simulink model "PV_MPPT_DesktopSim"  (R2025b)
settings: Solver=ode23t  StartTime=0.0  StopTime=inf  MaxStep=1e-4  RelTol=1e-3
PreLoadFcn:
  | load('EmulatedPV_LowPowerData.mat');
  | 
  | numIrr = 10;
  | ArrayPower = ArrayCurrent.*ArrayVoltage;
InitFcn:
  | Ts = 1e-4;
  | Tc = Ts;
undefined symbols (not defined in the file): ArrayCurrent, ArrayVoltage, DiscIntNeverNeededParam, Irradiance, Tdata
libraries: fl_lib x15, nesl_utility x9, ee_lib x2, slpidlib x2, eePwmGeneratorMultilevel x1, simulink x1, eePwmGenerator x1, eePowerMeasurement x1
settings Model: Creator=mmishra  LastModifiedBy=jlesage
settings SolverCC: AlgebraicLoopSolver=TrustRegion
settings DataIOCC: ReturnWorkspaceOutputs=off
settings DebuggingCC: UnconnectedInputMsg=warning  UnconnectedOutputMsg=warning  UnconnectedLineMsg=warning  ArithmeticOperatorsInVariantConditions=warning
settings ModelReferenceCC: EnableRefExpFcnMdlSchedulingChecks=on
settings SFSimCC: SimUseLocalCustomCode=off  CustomCodeUndefinedFunction=UseInterfaceOnly
settings RTWCC: RTWUseLocalCustomCode=off  GPUComputeCapability=3.5

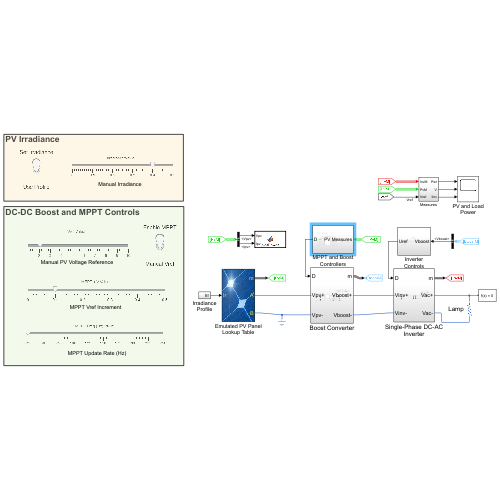
[thumbnail: Simulink's stored preview of the top-level diagram]
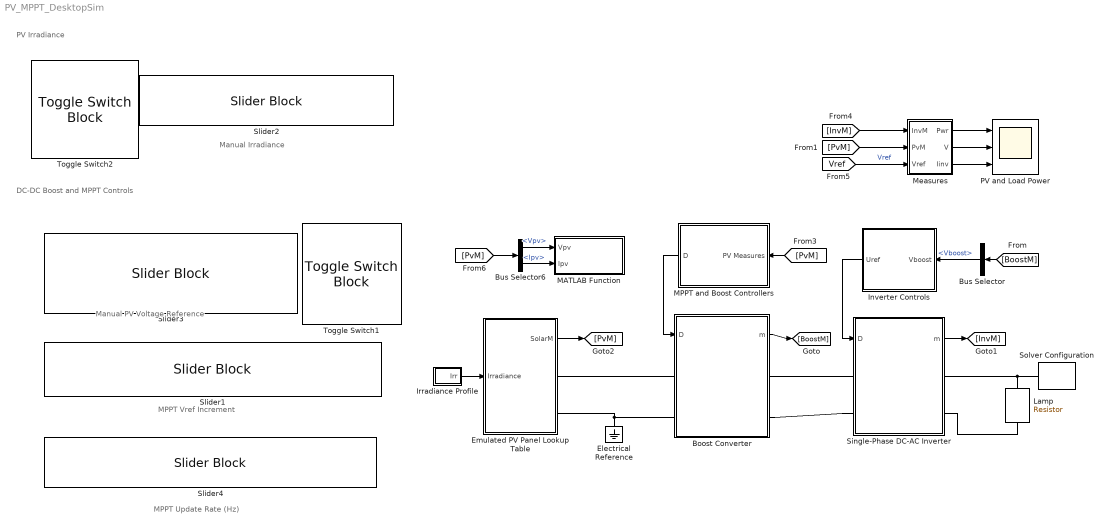
== system PV_MPPT_DesktopSim ==
  note: Manual Irradiance
  note: PV Irradiance
  note: MPPT Update Rate (Hz)
  note: MPPT Vref Increment
  note: DC-DC Boost and MPPT Controls
  note: Manual PV Voltage Reference
  Boost Converter : Subsystem
  Bus Selector : BusSelector  OutputSignals=Vboost
  Bus Selector6 : BusSelector  OutputSignals=Vpv,Ipv
  Electrical Reference : fl_lib/Electrical/Electrical Elements/Electrical Reference
  Emulated PV Panel Lookup Table : Subsystem
      mask Display:
      | image(imread('panel.jpg'))
      | color('yellow')
      | port_label('input',1,'Ir')
      | port_label('output',1,'m')
      | port_label('Rconn',1,'A')
      | port_label('Rconn',2,'B')
  Inverter Controls : Subsystem
  Irradiance Profile : Subsystem
  Lamp : fl_lib/Electrical/Electrical Elements/Resistor  R=11.5 Ohm  i_specify=off  i_priority=None  i=0 A  i_nominal_specify=off  i_nominal_value=1  i_nominal_unit=A  v_specify=off  v_priority=None  v=0 V  v_nominal_specify=off  v_nominal_value=1  v_nominal_unit=V
  MATLAB Function : MATLAB Function  TreatAsAtomicUnit=on  SystemSampleTime=1/10
  MPPT and Boost Controllers : Subsystem
  Measures : Subsystem
  PV and Load Power : Scope  NumInputPorts=3
      settings: ActiveDisplayYMinimum=-7.1500966536491433  ActiveDisplayYMaximum=64.3508698828423
  Single-Phase DC-AC Inverter : Subsystem
  Slider1 : SliderBlock  ScaleMax=0.5  TickInterval=0.10000000000000001
  Slider2 : SliderBlock  ScaleMax=0.5  TickInterval=0.10000000000000001
  Slider3 : SliderBlock  ScaleMin=1  ScaleMax=10  TickInterval=1
  Slider4 : SliderBlock  ScaleMin=25  ScaleMax=250  TickInterval=25
  Solver Configuration : nesl_utility/Solver Configuration  PhysicalDomain=network_engine_domain  SubClassName=solver  LeftPortType=input  RightPortType=generic  Tones=[]  Harmonics=[]  SimulateNoise=off  Profile=off  UseLocalSampling=off  EnableSwitchedLinearOptims=on  FrequencyDomain=off  UseCCode=off  RelTol=0.001  AbsTol=1e-06  MinStep=1e-09  ToWorkspace=off  RevertToSquareIcSolve=off  NumHomotopyIterations=100  PhasorMode=off  PhasorModeNumHarmonics=1  ConsistencySolver=NEWTON_FTOL  IndexReductionMethod=DerivativeReplacement  DoDC=off  ResidualTolerance=1e-09  ConsistencyTolSource=GLOBAL  ConsistencyAbsTol=0.001  ConsistencyRelTol=0.001  ConsistencyTolFactor=0.001  UseLocalSolver=on  LocalSolverChoice=NE_BACKWARD_EULER_ADVANCER  ResolveIndetEquations=on  FunctionEvalNumThread=1  LocalSolverSampleTime=Ts  DoFixedCost=on  MaxNonlinIter=3  MaxModeIter=2  ComputeImpulses=off  ImpulseIterations=2  LinearAlgebra=auto  LinearAlgebraNumThread=0  EquationFormulation=NE_TIME_EF  DelaysMemoryBudget=1024  AutomaticFiltering=on  FilteringTimeConstant=0.001  PartitionStorageMethod=AS_NEEDED  PartitionMemoryBudget=1024  PartitionMethod=ROBUST  MultibodyUseLocalSolver=off  MultibodyLocalSolverChoice=ODE1  MultibodyLocalSolverSampleTime=0.001
  Toggle Switch1 : ToggleSwitchBlock  LabelPosition=Hide
  Toggle Switch2 : ToggleSwitchBlock  LabelPosition=Hide
  wires:
  Irradiance Profile/1(Irr) -> Emulated PV Panel Lookup Table/1(Irradiance)
  Single-Phase DC-AC Inverter/1(m) -> [InvM]
  Emulated PV Panel Lookup Table/1(SolarM) -> [PvM]
  MPPT and Boost Controllers/1(D) -> Boost Converter/1(D)
  Boost Converter/1(m) -> [BoostM]
  [PvM] -> MPPT and Boost Controllers/1(PV Measures)
  Bus Selector/1 -> Inverter Controls/1(Vboost)  "<Vboost>"
  Inverter Controls/1(Uref) -> Single-Phase DC-AC Inverter/1(D)
  [BoostM] -> Bus Selector/1
  Bus Selector6/1 -> MATLAB Function/1(Vpv)  "<Vpv>"
  Bus Selector6/2 -> MATLAB Function/2(Ipv)  "<Ipv>"
  [PvM] -> Bus Selector6/1
  [InvM] -> Measures/1(InvM)
  [PvM] -> Measures/2(PvM)
  [Vref] -> Measures/3(Vref)  "Vref"
  Measures/1(Pwr) -> PV and Load Power/1
  Measures/2(V) -> PV and Load Power/2
  Measures/3(Iinv) -> PV and Load Power/3
  connections:
  Boost Converter/LConn1 -- Emulated PV Panel Lookup Table/RConn1
  Boost Converter/LConn2 -- Emulated PV Panel Lookup Table/RConn2 -- Electrical Reference/LConn1
  Lamp/LConn1 -- Solver Configuration/RConn1 -- Single-Phase DC-AC Inverter/RConn1
  Lamp/RConn1 -- Single-Phase DC-AC Inverter/RConn2
  Boost Converter/RConn1 -- Single-Phase DC-AC Inverter/LConn1
  Single-Phase DC-AC Inverter/LConn2 -- Boost Converter/RConn2

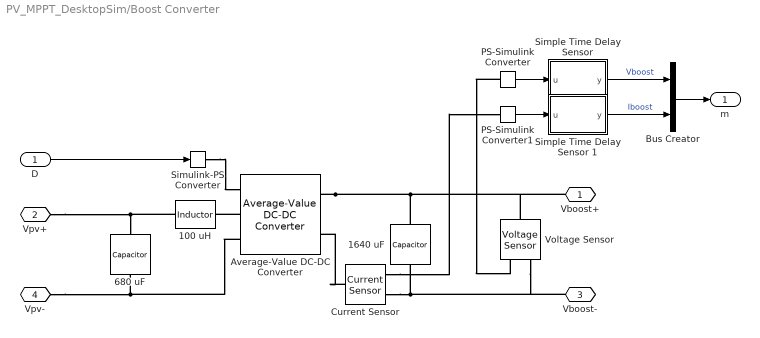
== system PV_MPPT_DesktopSim/Boost Converter ==
  D : Inport
  100 uH : fl_lib/Electrical/Electrical Elements/Inductor  l=100 uH  r=0 Ohm  g=0 1/Ohm  i_specify=off  i_priority=None  i=0 A  i_nominal_specify=off  i_nominal_value=1  i_nominal_unit=A  v_specify=off  v_priority=None  v=0 V  v_nominal_specify=off  v_nominal_value=1  v_nominal_unit=V  i_L_specify=off  i_L_priority=High  i_L=0 A  i_L_nominal_specify=off  i_L_nominal_value=1  i_L_nominal_unit=A
  1640 uF : fl_lib/Electrical/Electrical Elements/Capacitor  c=1640 uF  r=0 Ohm  g=0 1/Ohm  i_specify=off  i_priority=None  i=0 A  i_nominal_specify=off  i_nominal_value=1  i_nominal_unit=A  v_specify=off  v_priority=None  v=0 V  v_nominal_specify=off  v_nominal_value=1  v_nominal_unit=V  vc_specify=off  vc_priority=High  vc=0 V  vc_nominal_specify=off  vc_nominal_value=1  vc_nominal_unit=V
  680 uF : fl_lib/Electrical/Electrical Elements/Capacitor  c=680 uF  r=0 Ohm  g=0 1/Ohm  i_specify=off  i_priority=None  i=0 A  i_nominal_specify=off  i_nominal_value=1  i_nominal_unit=A  v_specify=off  v_priority=None  v=0 V  v_nominal_specify=off  v_nominal_value=1  v_nominal_unit=V  vc_specify=off  vc_priority=High  vc=0 V  vc_nominal_specify=off  vc_nominal_value=1  vc_nominal_unit=V
  Average-Value DC-DC Converter : ee_lib/Semiconductors & Converters/Converters/Average-Value DC-DC Converter  implementation_option=ee.enum.converters.implementation.behavioral  converter_type=ee.enum.converters.dcdctype.boost  control_option=ee.enum.converters.controlinput.dutycycle  efficiency_option=ee.enum.converters.efficiency.constant  efficiency_fixed=100  i_vec=[0, 2, 5] A  efficiency_vec=[90, 95, 98]  Lf=1e-6 H  Rl=0 Ohm  Cf=1e-7 F  Rc=1e-6 Ohm  iL_specify=off  iL_priority=High  iL=0 A  iL_nominal_specify=off  iL_nominal_value=1  iL_nominal_unit=A  vc_specify=off  vc_priority=High  vc=0 V  vc_nominal_specify=off  vc_nominal_value=1  vc_nominal_unit=V
      settings: InternalSimscapePortConfiguration="{\"Bottom\":[],\"Left\":[{\"id\":\"DutyCycle\",\"label\":\"DutyCycle\",\"type\":\"input\"},{\"id\":\"p1\",\"label\":\"1+\",\"type\":\"foundation.electrical.electrical\"},{\"id\":\"n1\",\"label\":\"1-\",\"type\":\"foundation.electrical.electrical\"}],\"Right\":[{\"id\":\"p2\",\"label\":\"2+\",\"type\":\"foundation.electrical.electrical\"},{\"id\":\"n2\",\"label\":\"2-\",\"type\":\"foundation.electrical.electrical\"}],\"Top\":[]}"
  Bus Creator : BusCreator  Inputs=2
  Current Sensor : fl_lib/Electrical/Electrical Sensors/Current Sensor
  PS-Simulink Converter : nesl_utility/PS-Simulink Converter  PhysicalDomain=network_engine_domain  SubClassName=ps_output  LeftPortType=input  RightPortType=output  PseudoPeriodic=off  Frequencies=[]  VectorFormat=1-D array  Unit=inherit  AffineConversion=off
  PS-Simulink Converter1 : nesl_utility/PS-Simulink Converter  PhysicalDomain=network_engine_domain  SubClassName=ps_output  LeftPortType=input  RightPortType=output  PseudoPeriodic=off  Frequencies=[]  VectorFormat=1-D array  Unit=inherit  AffineConversion=off
  "Simple Time Delay Sensor " : Subsystem  mask{Ts=Ts, Tau=0.0001}
      mask prompts: Ts "Sample Time, [s]"; Tau "Time Constant, Tau [s]"
      mask help: Simple Sensor
      mask Display: fprintf('1\n------------\n(1 + s Tau)');
  Simple Time Delay Sensor 1 : Subsystem  mask{Ts=Ts, Tau=0.0001}
      mask prompts: Ts "Sample Time, [s]"; Tau "Time Constant, Tau [s]"
      mask help: Simple Sensor
      mask Display: fprintf('1\n------------\n(1 + s Tau)');
  Simulink-PS Converter : nesl_utility/Simulink-PS Converter  PhysicalDomain=network_engine_domain  SubClassName=ps_input  LeftPortType=input  RightPortType=output  PseudoPeriodic=off  Frequencies=[]  NoiseDistribution=none  NoiseParameters=[]  Unit=1  AffineConversion=off  FilteringAndDerivatives=filter  SimscapeFilterOrder=2  InputFilterTimeConstant=0.001  UdotUserProvided=0
  Voltage Sensor : fl_lib/Electrical/Electrical Sensors/Voltage Sensor
  Vboost+ : PMIOPort  Side=Right
  Vpv+ : PMIOPort  Port=2  Side=Left
  Vboost- : PMIOPort  Port=3  Side=Right
  Vpv- : PMIOPort  Port=4  Side=Left
  m : Outport  VectorParamsAs1DForOutWhenUnconnected=off
  wires:
  D/1 -> Simulink-PS Converter/1
  "Simple Time Delay Sensor "/1(y) -> Bus Creator/1  "Vboost"
  Bus Creator/1 -> m/1
  Simple Time Delay Sensor 1/1(y) -> Bus Creator/2  "Iboost"
  PS-Simulink Converter/1 -> "Simple Time Delay Sensor "/1(u)
  PS-Simulink Converter1/1 -> Simple Time Delay Sensor 1/1(u)
  connections:
  Current Sensor/RConn2 -- 1640 uF/RConn1 -- Vboost-/RConn1 -- Voltage Sensor/RConn2
  Vpv-/RConn1 -- Average-Value DC-DC Converter/LConn3 -- 680 uF/RConn1
  Average-Value DC-DC Converter/LConn2 -- 100 uH/RConn1
  Simulink-PS Converter/RConn1 -- Average-Value DC-DC Converter/LConn1
  Average-Value DC-DC Converter/RConn1 -- 1640 uF/LConn1 -- Voltage Sensor/LConn1 -- Vboost+/RConn1
  100 uH/LConn1 -- 680 uF/LConn1 -- Vpv+/RConn1
  PS-Simulink Converter/LConn1 -- Voltage Sensor/RConn1
  Current Sensor/LConn1 -- Average-Value DC-DC Converter/RConn2
  Current Sensor/RConn1 -- PS-Simulink Converter1/LConn1

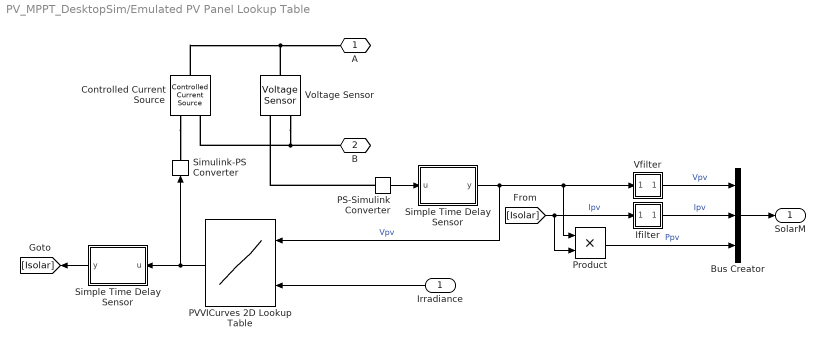
== system PV_MPPT_DesktopSim/Emulated PV Panel Lookup Table ==
  Irradiance : Inport
  Bus Creator : BusCreator  Inputs=3
  Controlled Current Source : fl_lib/Electrical/Electrical Sources/Controlled Current Source
  Ifilter : Subsystem  mask{Tf=0.01}
      mask prompts: Tf "Filter Time Constant"
  PS-Simulink Converter : nesl_utility/PS-Simulink Converter  PhysicalDomain=network_engine_domain  SubClassName=ps_output  LeftPortType=input  RightPortType=output  PseudoPeriodic=off  Frequencies=[]  VectorFormat=1-D array  Unit=inherit  AffineConversion=off
  PVVICurves 2D Lookup Table : Lookup_n-D  BreakpointsForDimension1=ArrayVoltage  BreakpointsForDimension2=Irradiance  Table=ArrayCurrent  InternalRulePriority=Speed  RndMeth=Simplest
      settings: InputPortMap=u0,u1
  Product : Product
  Simple Time Delay Sensor : Subsystem  mask{Ts=Ts, Tau=0.0001}
      mask prompts: Ts "Sample Time, [s]"; Tau "Time Constant, Tau [s]"
      mask help: Simple Sensor
      mask Display: fprintf('1\n------------\n(1 + s Tau)');
  "Simple Time Delay Sensor " : Subsystem  mask{Ts=Ts, Tau=0.0001}
      mask prompts: Ts "Sample Time, [s]"; Tau "Time Constant, Tau [s]"
      mask help: Simple Sensor
      mask Display: fprintf('1\n------------\n(1 + s Tau)');
  Simulink-PS Converter : nesl_utility/Simulink-PS Converter  PhysicalDomain=network_engine_domain  SubClassName=ps_input  LeftPortType=input  RightPortType=output  PseudoPeriodic=off  Frequencies=[]  NoiseDistribution=none  NoiseParameters=[]  Unit=1  AffineConversion=off  FilteringAndDerivatives=filter  SimscapeFilterOrder=2  InputFilterTimeConstant=0.001  UdotUserProvided=0
  Vfilter : Subsystem  mask{Tf=0.01}
      mask prompts: Tf "Filter Time Constant"
  Voltage Sensor : fl_lib/Electrical/Electrical Sensors/Voltage Sensor
  A : PMIOPort  Side=Right
  B : PMIOPort  Port=2  Side=Right
  SolarM : Outport  VectorParamsAs1DForOutWhenUnconnected=off
  wires:
  Irradiance/1 -> PVVICurves 2D Lookup Table/2
  PVVICurves 2D Lookup Table/1 -> Simple Time Delay Sensor/1(u), Simulink-PS Converter/1
  Bus Creator/1 -> SolarM/1
  [Isolar] -> Product/2, Ifilter/1(u)  "Ipv"
  Product/1 -> Bus Creator/3  "Ppv"
  Simple Time Delay Sensor/1(y) -> [Isolar]
  "Simple Time Delay Sensor "/1(y) -> Product/1, Vfilter/1(u), PVVICurves 2D Lookup Table/1  "Vpv"
  PS-Simulink Converter/1 -> "Simple Time Delay Sensor "/1(u)
  Vfilter/1(y) -> Bus Creator/1  "Vpv"
  Ifilter/1(y) -> Bus Creator/2  "Ipv"
  connections:
  Controlled Current Source/LConn1 -- Voltage Sensor/LConn1 -- A/RConn1
  B/RConn1 -- Voltage Sensor/RConn2 -- Controlled Current Source/RConn2
  Controlled Current Source/RConn1 -- Simulink-PS Converter/RConn1
  PS-Simulink Converter/LConn1 -- Voltage Sensor/RConn1

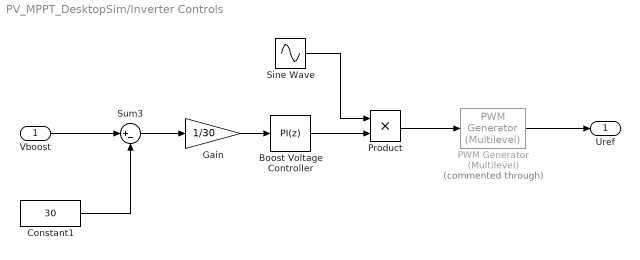
== system PV_MPPT_DesktopSim/Inverter Controls ==
  Vboost : Inport
  Boost Voltage Controller : slpidlib/PID Controller  Controller=PI  Form=Parallel  TimeDomain=Discrete-time  UseExternalTs=off  SampleTime=Tc  IntegratorMethod=Forward Euler  FilterMethod=Forward Euler  ControllerParametersSource=internal  P=3  I=250  UseKiTs=off  D=0  UseExternalDerivativeSource=off  N=100  UseFilter=on  TunerSelectOption=Transfer Function Based (PID Tuner App)  InitialConditionSource=internal  InitialConditionForIntegrator=1  InitialConditionForFilter=0  DifferentiatorICPrevScaledInput=0  ExternalReset=none  TrackingMode=off  Kt=1  LimitOutput=on  SatLimitsSource=internal  UpperSaturationLimit=1  LowerSaturationLimit=0  LinearizeAsGain=on  AntiWindupMode=clamping  Kb=1  LimitIntegrator=off  UpperIntegratorSaturationLimit=inf  LowerIntegratorSaturationLimit=-inf  POutMin=[]  POutMax=[]  IOutMin=[]  IOutMax=[]  DOutMin=[]  DOutMax=[]  NOutMin=[]  NOutMax=[]  SumOutMin=[]  SumOutMax=[]  SaturationOutMin=[]  SaturationOutMax=[]  PParamMin=[]  PParamMax=[]  IParamMin=[]  IParamMax=[]  DParamMin=[]  DParamMax=[]  NParamMin=[]  NParamMax=[]  KbParamMin=[]  KbParamMax=[]  KtParamMin=[]  KtParamMax=[]  KbOutMin=[]  KbOutMax=[]  KtOutMin=[]  KtOutMax=[]  IntegratorOutMin=[]  IntegratorOutMax=[]  FilterOutMin=[]  FilterOutMax=[]  SumI1OutMin=[]  SumI1OutMax=[]  SumI2OutMin=[]  SumI2OutMax=[]  SumI3OutMin=[]  SumI3OutMax=[]  SumI4OutMin=[]  SumI4OutMax=[]  SumDOutMin=[]  SumDOutMax=[]  DifferentiatorOutMin=[]  DifferentiatorOutMax=[]  FilterDiffOutCoefMin=[]  FilterDiffOutCoefMax=[]  ReciprocalOutMin=[]  ReciprocalOutMax=[]  SumDenOutMin=[]  SumDenOutMax=[]  SumNumOutMin=[]  SumNumOutMax=[]  DivideOutMin=[]  DivideOutMax=[]  UdiffTsProdOutMin=[]  UdiffTsProdOutMax=[]  NTsProdOutMin=[]  NTsProdOutMax=[]  UintegralTsProdOutMin=[]  UintegralTsProdOutMax=[]  UngainTsProdOutMin=[]  UngainTsProdOutMax=[]  ClampingZeroOutDataTypeStr=Inherit: Inherit via back propagation  ClampingZeroOutMin=[]  ClampingZeroOutMax=[]  FilterDenConstantOutDataTypeStr=Inherit: Inherit via back propagation  FilterDenConstantOutMin=[]  FilterDenConstantOutMax=[]  PCopyOutDataTypeStr=Inherit: Inherit via back propagation  PCopyOutMin=[]  PCopyOutMax=[]  NCopyOutDataTypeStr=Inherit: Inherit via back propagation  NCopyOutMin=[]  NCopyOutMax=[]  IntegratorContinuousStateAttributes=''  IntegratorStateMustResolveToSignalObject=off  IntegratorRTWStateStorageClass=Auto  FilterContinuousStateAttributes=''  FilterStateMustResolveToSignalObject=off  FilterRTWStateStorageClass=Auto  ParallelPVariant=InternalParameters  IdealPVariant=Disabled  IVariant=InternalParameters  DVariant=Disabled  IntegratorVariant=Discrete  SatVariant=Enabled  AWVariant=DiscClampingParallel  PCopyVariant=Disabled  TRVariant=Disabled  FdbkBlocksVariant=Forward  IdealPFdbkVariant=Disabled  SatFdbkVariant=Disabled  DerivativeFilterVariant=Disabled  NVariant=Disabled  NCopyVariant=Disabled_SignalSpec  FilterICVariant=Disabled  IntegratorICVariant=InternalICs  ExternalResetVariant=Disabled  TRSumVariant=Passthrough  SumFdbkVariant=Disabled  SumVariant=Sum_PI  TsampFilterVariant=InternalTs  TsampNgainVariant=Passthrough  TsampIntegralVariant=Disabled_SignalSpec  ExternalSaturationOutDataTypeStr=Inherit: Same as second input  DerivativeSourceVariant=Disabled  PreIntVariant=InternalPreInt
  Constant1 : Constant  Value=30
  Gain : Gain  Gain=1/30
  PWM Generator (Multilevel) : eePwmGeneratorMultilevel/PWM Generator (Multilevel)  Commented=through  topology=Full-bridge  Nsm=1  Tper=1/6000  Ts=Ts
      settings: LibrarySourceBlock=|
      | ee_sl_lib/Pulse Width
      | Modulation/PWM Generator
      | (Multilevel)
  Product : Product
  Sine Wave : Sin  Frequency=2*pi*60  SampleTime=Tc
  Sum3 : Sum  Inputs=|+-
  Uref : Outport  VectorParamsAs1DForOutWhenUnconnected=off
  wires:
  Constant1/1 -> Sum3/2
  Sine Wave/1 -> Product/1
  Boost Voltage Controller/1 -> Product/2
  Sum3/1 -> Gain/1
  Vboost/1 -> Sum3/1
  Gain/1 -> Boost Voltage Controller/1
  Product/1 -> PWM Generator (Multilevel)/1
  PWM Generator (Multilevel)/1 -> Uref/1

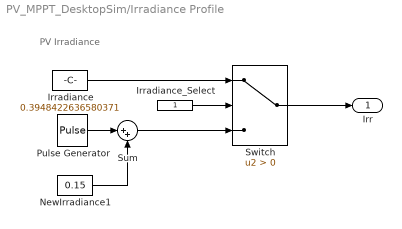
== system PV_MPPT_DesktopSim/Irradiance Profile ==
  note: PV Irradiance
  Irradiance : Constant  Value=0.3948422636580371  OutDataTypeStr=single
  Irradiance_Select : Constant  OutDataTypeStr=single
  NewIrradiance1 : Constant  Value=0.15  OutDataTypeStr=single
  Pulse Generator : DiscretePulseGenerator  PulseType=Time based  Amplitude=0.15  Period=10  PulseWidth=50
  Sum : Sum  Inputs=|++
  Switch : Switch  Criteria=u2 > Threshold  SaturateOnIntegerOverflow=off  InputSameDT=off
  Irr : Outport  VectorParamsAs1DForOutWhenUnconnected=off
  wires:
  NewIrradiance1/1 -> Sum/2
  Pulse Generator/1 -> Sum/1
  Sum/1 -> Switch/3
  Irradiance/1 -> Switch/1
  Switch/1 -> Irr/1
  Irradiance_Select/1 -> Switch/2

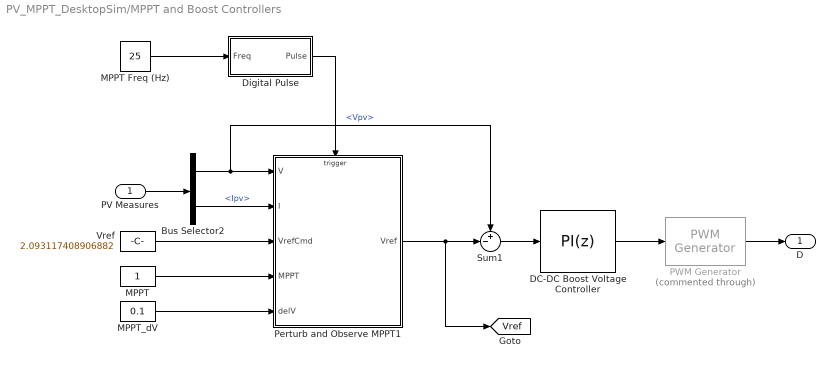
== system PV_MPPT_DesktopSim/MPPT and Boost Controllers ==
  PV Measures : Inport
  Bus Selector2 : BusSelector  OutputSignals=Vpv,Ipv
  DC-DC Boost Voltage Controller : slpidlib/PID Controller  Controller=PI  Form=Parallel  TimeDomain=Discrete-time  UseExternalTs=off  SampleTime=Tc  IntegratorMethod=Forward Euler  FilterMethod=Forward Euler  ControllerParametersSource=internal  P=0.015  I=2.5  UseKiTs=off  D=0  UseExternalDerivativeSource=off  N=100  UseFilter=on  TunerSelectOption=Transfer Function Based (PID Tuner App)  InitialConditionSource=internal  InitialConditionForIntegrator=0  InitialConditionForFilter=0  DifferentiatorICPrevScaledInput=0  ExternalReset=none  TrackingMode=off  Kt=1  LimitOutput=on  SatLimitsSource=internal  UpperSaturationLimit=1  LowerSaturationLimit=0  LinearizeAsGain=on  AntiWindupMode=clamping  Kb=1  LimitIntegrator=off  UpperIntegratorSaturationLimit=inf  LowerIntegratorSaturationLimit=-inf  POutMin=[]  POutMax=[]  IOutMin=[]  IOutMax=[]  DOutMin=[]  DOutMax=[]  NOutMin=[]  NOutMax=[]  SumOutMin=[]  SumOutMax=[]  SaturationOutMin=[]  SaturationOutMax=[]  PParamMin=[]  PParamMax=[]  IParamMin=[]  IParamMax=[]  DParamMin=[]  DParamMax=[]  NParamMin=[]  NParamMax=[]  KbParamMin=[]  KbParamMax=[]  KtParamMin=[]  KtParamMax=[]  KbOutMin=[]  KbOutMax=[]  KtOutMin=[]  KtOutMax=[]  IntegratorOutMin=[]  IntegratorOutMax=[]  FilterOutMin=[]  FilterOutMax=[]  SumI1OutMin=[]  SumI1OutMax=[]  SumI2OutMin=[]  SumI2OutMax=[]  SumI3OutMin=[]  SumI3OutMax=[]  SumI4OutMin=[]  SumI4OutMax=[]  SumDOutMin=[]  SumDOutMax=[]  DifferentiatorOutMin=[]  DifferentiatorOutMax=[]  FilterDiffOutCoefMin=[]  FilterDiffOutCoefMax=[]  ReciprocalOutMin=[]  ReciprocalOutMax=[]  SumDenOutMin=[]  SumDenOutMax=[]  SumNumOutMin=[]  SumNumOutMax=[]  DivideOutMin=[]  DivideOutMax=[]  UdiffTsProdOutMin=[]  UdiffTsProdOutMax=[]  NTsProdOutMin=[]  NTsProdOutMax=[]  UintegralTsProdOutMin=[]  UintegralTsProdOutMax=[]  UngainTsProdOutMin=[]  UngainTsProdOutMax=[]  ClampingZeroOutDataTypeStr=Inherit: Inherit via back propagation  ClampingZeroOutMin=[]  ClampingZeroOutMax=[]  FilterDenConstantOutDataTypeStr=Inherit: Inherit via back propagation  FilterDenConstantOutMin=[]  FilterDenConstantOutMax=[]  PCopyOutDataTypeStr=Inherit: Inherit via back propagation  PCopyOutMin=[]  PCopyOutMax=[]  NCopyOutDataTypeStr=Inherit: Inherit via back propagation  NCopyOutMin=[]  NCopyOutMax=[]  IntegratorContinuousStateAttributes=''  IntegratorStateMustResolveToSignalObject=off  IntegratorRTWStateStorageClass=Auto  FilterContinuousStateAttributes=''  FilterStateMustResolveToSignalObject=off  FilterRTWStateStorageClass=Auto  ParallelPVariant=InternalParameters  IdealPVariant=Disabled  IVariant=InternalParameters  DVariant=Disabled  IntegratorVariant=Discrete  SatVariant=Enabled  AWVariant=DiscClampingParallel  PCopyVariant=Disabled  TRVariant=Disabled  FdbkBlocksVariant=Forward  IdealPFdbkVariant=Disabled  SatFdbkVariant=Disabled  DerivativeFilterVariant=Disabled  NVariant=Disabled  NCopyVariant=Disabled_SignalSpec  FilterICVariant=Disabled  IntegratorICVariant=InternalICs  ExternalResetVariant=Disabled  TRSumVariant=Passthrough  SumFdbkVariant=Disabled  SumVariant=Sum_PI  TsampFilterVariant=InternalTs  TsampNgainVariant=Passthrough  TsampIntegralVariant=Disabled_SignalSpec  ExternalSaturationOutDataTypeStr=Inherit: Same as second input  DerivativeSourceVariant=Disabled  PreIntVariant=InternalPreInt
  Digital Pulse : Subsystem  mask{Ts=Tc, Duty=0.5}
      mask prompts: Ts "Sample Rate [s]"; Duty "Duty Cycle [0-1]"
  MPPT : Constant
  MPPT Freq (Hz) : Constant  Value=25
  MPPT_dV : Constant  Value=0.1
  PWM Generator : eePwmGenerator/PWM Generator  Commented=through  CarrCount=Up  Tper=1/5000  Tdelay=0  Ts=Ts
  Perturb and Observe MPPT1 : Stateflow chart  TreatAsAtomicUnit=on  SystemSampleTime=Tdata
  Sum1 : Sum  Inputs=+-|
  Vref : Constant  Value=2.093117408906882
  D : Outport  VectorParamsAs1DForOutWhenUnconnected=off
  tag scope: Vref=global
  wires:
  PV Measures/1 -> Bus Selector2/1
  Digital Pulse/1(Pulse) -> Perturb and Observe MPPT1/Trigger
  MPPT Freq (Hz)/1 -> Digital Pulse/1(Freq)
  MPPT_dV/1 -> Perturb and Observe MPPT1/5(delV)
  Vref/1 -> Perturb and Observe MPPT1/3(VrefCmd)
  Sum1/1 -> DC-DC Boost Voltage Controller/1
  MPPT/1 -> Perturb and Observe MPPT1/4(MPPT)
  Bus Selector2/1 -> Perturb and Observe MPPT1/1(V), Sum1/1  "<Vpv>"
  Perturb and Observe MPPT1/1(Vref) -> [Vref], Sum1/2
  Bus Selector2/2 -> Perturb and Observe MPPT1/2(I)  "<Ipv>"
  DC-DC Boost Voltage Controller/1 -> PWM Generator/1
  PWM Generator/1 -> D/1

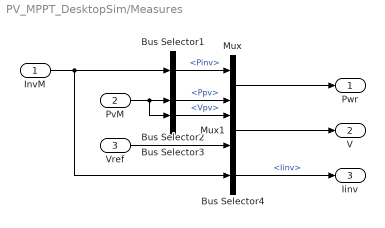
== system PV_MPPT_DesktopSim/Measures ==
  InvM : Inport
  PvM : Inport  Port=2
  Vref : Inport  Port=3
  Bus Selector1 : BusSelector  OutputSignals=Pinv
  Bus Selector2 : BusSelector  OutputSignals=Ppv
  Bus Selector3 : BusSelector  OutputSignals=Vpv
  Bus Selector4 : BusSelector  OutputSignals=Iinv
  Mux : Mux  Inputs=2
  Mux1 : Mux  Inputs=2
  Pwr : Outport  VectorParamsAs1DForOutWhenUnconnected=off
  V : Outport  Port=2  VectorParamsAs1DForOutWhenUnconnected=off
  Iinv : Outport  Port=3  VectorParamsAs1DForOutWhenUnconnected=off
  wires:
  Bus Selector2/1 -> Mux/2  "<Ppv>"
  PvM/1 -> Bus Selector3/1, Bus Selector2/1
  Mux/1 -> Pwr/1
  Bus Selector1/1 -> Mux/1  "<Pinv>"
  Bus Selector3/1 -> Mux1/1  "<Vpv>"
  Bus Selector4/1 -> Iinv/1  "<Iinv>"
  Mux1/1 -> V/1
  Vref/1 -> Mux1/2
  InvM/1 -> Bus Selector4/1, Bus Selector1/1

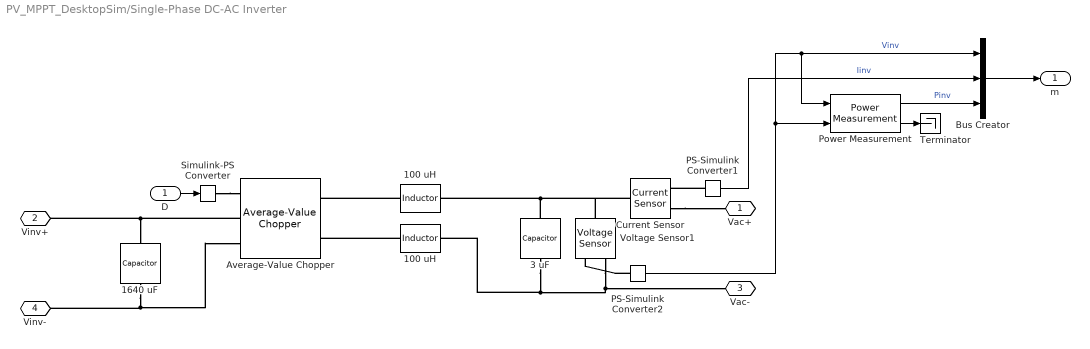
== system PV_MPPT_DesktopSim/Single-Phase DC-AC Inverter ==
  D : Inport
  100 uH : fl_lib/Electrical/Electrical Elements/Inductor  l=100 uH  r=0 Ohm  g=0 1/Ohm  i_specify=off  i_priority=None  i=0 A  i_nominal_specify=off  i_nominal_value=1  i_nominal_unit=A  v_specify=off  v_priority=None  v=0 V  v_nominal_specify=off  v_nominal_value=1  v_nominal_unit=V  i_L_specify=off  i_L_priority=High  i_L=0 A  i_L_nominal_specify=off  i_L_nominal_value=1  i_L_nominal_unit=A
  "100 uH " : fl_lib/Electrical/Electrical Elements/Inductor  l=100 uH  r=0 Ohm  g=0 1/Ohm  i_specify=off  i_priority=None  i=0 A  i_nominal_specify=off  i_nominal_value=1  i_nominal_unit=A  v_specify=off  v_priority=None  v=0 V  v_nominal_specify=off  v_nominal_value=1  v_nominal_unit=V  i_L_specify=off  i_L_priority=High  i_L=0 A  i_L_nominal_specify=off  i_L_nominal_value=1  i_L_nominal_unit=A
  1640 uF : fl_lib/Electrical/Electrical Elements/Capacitor  c=1640 uF  r=0.05 Ohm  g=0 1/Ohm  i_specify=off  i_priority=None  i=0 A  i_nominal_specify=off  i_nominal_value=1  i_nominal_unit=A  v_specify=off  v_priority=None  v=0 V  v_nominal_specify=off  v_nominal_value=1  v_nominal_unit=V  vc_specify=off  vc_priority=High  vc=0 V  vc_nominal_specify=off  vc_nominal_value=1  vc_nominal_unit=V
  3 uF : fl_lib/Electrical/Electrical Elements/Capacitor  c=3 uF  r=0 Ohm  g=0 1/Ohm  i_specify=off  i_priority=None  i=0 A  i_nominal_specify=off  i_nominal_value=1  i_nominal_unit=A  v_specify=off  v_priority=None  v=0 V  v_nominal_specify=off  v_nominal_value=1  v_nominal_unit=V  vc_specify=off  vc_priority=High  vc=0 V  vc_nominal_specify=off  vc_nominal_value=1  vc_nominal_unit=V
  Average-Value Chopper : ee_lib/Semiconductors & Converters/Converters/Average-Value Chopper  chopper_type=5  efficiency_option=1  efficiency_fixed=100  i_vec=[0, 2, 5] A  efficiency_vec=[90, 95, 98]
      settings: InternalSimscapePortConfiguration="{\"Bottom\":[],\"Left\":[{\"id\":\"DutyCycle\",\"label\":\"DutyCycle\",\"type\":\"input\"},{\"id\":\"p1\",\"label\":\"1+\",\"type\":\"foundation.electrical.electrical\"},{\"id\":\"n1\",\"label\":\"1-\",\"type\":\"foundation.electrical.electrical\"}],\"Right\":[{\"id\":\"p2\",\"label\":\"2+\",\"type\":\"foundation.electrical.electrical\"},{\"id\":\"n2\",\"label\":\"2-\",\"type\":\"foundation.electrical.electrical\"}],\"Top\":[]}"
  Bus Creator : BusCreator  Inputs=3
  Current Sensor : fl_lib/Electrical/Electrical Sensors/Current Sensor
  PS-Simulink Converter1 : nesl_utility/PS-Simulink Converter  PhysicalDomain=network_engine_domain  SubClassName=ps_output  LeftPortType=input  RightPortType=output  PseudoPeriodic=off  Frequencies=[]  VectorFormat=1-D array  Unit=inherit  AffineConversion=off
  PS-Simulink Converter2 : nesl_utility/PS-Simulink Converter  PhysicalDomain=network_engine_domain  SubClassName=ps_output  LeftPortType=input  RightPortType=output  PseudoPeriodic=off  Frequencies=[]  VectorFormat=1-D array  Unit=inherit  AffineConversion=off
  Power Measurement : eePowerMeasurement/Power Measurement  LabelModeActiveChoice=Discrete  F=60  K=[0]  Ts=Ts
  Simulink-PS Converter : nesl_utility/Simulink-PS Converter  PhysicalDomain=network_engine_domain  SubClassName=ps_input  LeftPortType=input  RightPortType=output  PseudoPeriodic=off  Frequencies=[]  NoiseDistribution=none  NoiseParameters=[]  Unit=1  AffineConversion=off  FilteringAndDerivatives=filter  SimscapeFilterOrder=2  InputFilterTimeConstant=0.001  UdotUserProvided=0
  Terminator : Terminator
  Voltage Sensor1 : fl_lib/Electrical/Electrical Sensors/Voltage Sensor
  Vac+ : PMIOPort  Side=Right
  Vinv+ : PMIOPort  Port=2  Side=Left
  Vac- : PMIOPort  Port=3  Side=Right
  Vinv- : PMIOPort  Port=4  Side=Left
  m : Outport  VectorParamsAs1DForOutWhenUnconnected=off
  wires:
  Power Measurement/2 -> Terminator/1
  Power Measurement/1 -> Bus Creator/3  "Pinv"
  PS-Simulink Converter1/1 -> Bus Creator/2  "Iinv"
  PS-Simulink Converter2/1 -> Power Measurement/2, Power Measurement/1, Bus Creator/1  "Vinv"
  Bus Creator/1 -> m/1
  D/1 -> Simulink-PS Converter/1
  connections:
  PS-Simulink Converter1/LConn1 -- Current Sensor/RConn1
  3 uF/LConn1 -- 100 uH/RConn1 -- Current Sensor/LConn1 -- Voltage Sensor1/LConn1
  PS-Simulink Converter2/LConn1 -- Voltage Sensor1/RConn1
  3 uF/RConn1 -- "100 uH "/RConn1 -- Voltage Sensor1/RConn2 -- Vac-/RConn1
  Simulink-PS Converter/RConn1 -- Average-Value Chopper/LConn1
  Average-Value Chopper/LConn2 -- 1640 uF/LConn1 -- Vinv+/RConn1
  1640 uF/RConn1 -- Vinv-/RConn1 -- Average-Value Chopper/LConn3
  "100 uH "/LConn1 -- Average-Value Chopper/RConn2
  100 uH/LConn1 -- Average-Value Chopper/RConn1
  Current Sensor/RConn2 -- Vac+/RConn1

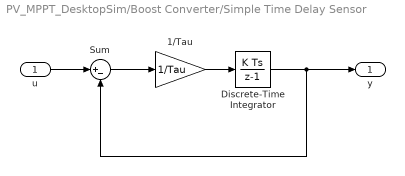
== system PV_MPPT_DesktopSim/Boost Converter/Simple Time Delay Sensor  ==
  u : Inport
  1/Tau : Gain  Gain=1/Tau
  Discrete-Time Integrator : DiscreteIntegrator  SampleTime=Ts  ICPrevOutput=DiscIntNeverNeededParam  ICPrevScaledInput=DiscIntNeverNeededParam
  Sum : Sum  Inputs=|+-
  y : Outport  VectorParamsAs1DForOutWhenUnconnected=off
  wires:
  Discrete-Time Integrator/1 -> Sum/2, y/1
  u/1 -> Sum/1
  Sum/1 -> 1/Tau/1
  1/Tau/1 -> Discrete-Time Integrator/1

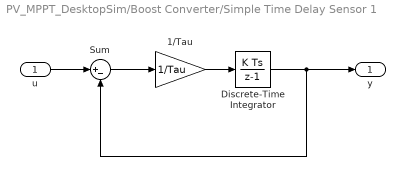
== system PV_MPPT_DesktopSim/Boost Converter/Simple Time Delay Sensor 1 ==
  u : Inport
  1/Tau : Gain  Gain=1/Tau
  Discrete-Time Integrator : DiscreteIntegrator  SampleTime=Ts  ICPrevOutput=DiscIntNeverNeededParam  ICPrevScaledInput=DiscIntNeverNeededParam
  Sum : Sum  Inputs=|+-
  y : Outport  VectorParamsAs1DForOutWhenUnconnected=off
  wires:
  1/Tau/1 -> Discrete-Time Integrator/1
  Sum/1 -> 1/Tau/1
  u/1 -> Sum/1
  Discrete-Time Integrator/1 -> y/1, Sum/2

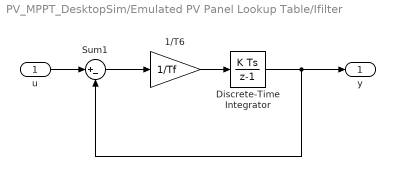
== system PV_MPPT_DesktopSim/Emulated PV Panel Lookup Table/Ifilter ==
  u : Inport
  1/T6 : Gain  Gain=1/Tf
  Discrete-Time Integrator : DiscreteIntegrator  SampleTime=Tc  ICPrevOutput=DiscIntNeverNeededParam  ICPrevScaledInput=DiscIntNeverNeededParam
  Sum1 : Sum  Inputs=|+-
  y : Outport  VectorParamsAs1DForOutWhenUnconnected=off
  wires:
  Sum1/1 -> 1/T6/1
  Discrete-Time Integrator/1 -> Sum1/2, y/1
  u/1 -> Sum1/1
  1/T6/1 -> Discrete-Time Integrator/1

== system PV_MPPT_DesktopSim/Emulated PV Panel Lookup Table/Simple Time Delay Sensor ==
  u : Inport
  1/Tau : Gain  Gain=1/Tau
  Discrete-Time Integrator : DiscreteIntegrator  SampleTime=Ts  ICPrevOutput=DiscIntNeverNeededParam  ICPrevScaledInput=DiscIntNeverNeededParam
  Sum : Sum  Inputs=|+-
  y : Outport  VectorParamsAs1DForOutWhenUnconnected=off
  wires:
  1/Tau/1 -> Discrete-Time Integrator/1
  Sum/1 -> 1/Tau/1
  u/1 -> Sum/1
  Discrete-Time Integrator/1 -> y/1, Sum/2

== system PV_MPPT_DesktopSim/Emulated PV Panel Lookup Table/Simple Time Delay Sensor  ==
  u : Inport
  1/Tau : Gain  Gain=1/Tau
  Discrete-Time Integrator : DiscreteIntegrator  SampleTime=Ts  ICPrevOutput=DiscIntNeverNeededParam  ICPrevScaledInput=DiscIntNeverNeededParam
  Sum : Sum  Inputs=|+-
  y : Outport  VectorParamsAs1DForOutWhenUnconnected=off
  wires:
  Discrete-Time Integrator/1 -> Sum/2, y/1
  u/1 -> Sum/1
  Sum/1 -> 1/Tau/1
  1/Tau/1 -> Discrete-Time Integrator/1

== system PV_MPPT_DesktopSim/Emulated PV Panel Lookup Table/Vfilter ==
  u : Inport
  1/T6 : Gain  Gain=1/Tf
  Discrete-Time Integrator : DiscreteIntegrator  SampleTime=Tc  ICPrevOutput=DiscIntNeverNeededParam  ICPrevScaledInput=DiscIntNeverNeededParam
  Sum1 : Sum  Inputs=|+-
  y : Outport  VectorParamsAs1DForOutWhenUnconnected=off
  wires:
  1/T6/1 -> Discrete-Time Integrator/1
  u/1 -> Sum1/1
  Discrete-Time Integrator/1 -> y/1, Sum1/2
  Sum1/1 -> 1/T6/1

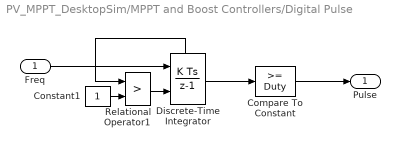
== system PV_MPPT_DesktopSim/MPPT and Boost Controllers/Digital Pulse ==
  Freq : Inport
  Compare To Constant : simulink/Logic and Bit Operations/Compare To Constant  relop=>=  const=Duty  OutDataTypeStr=boolean
  Constant1 : Constant
  Discrete-Time Integrator : DiscreteIntegrator  ExternalReset=rising  SampleTime=Ts  ShowStatePort=on  ICPrevOutput=DiscIntNeverNeededParam  ICPrevScaledInput=DiscIntNeverNeededParam
  Relational Operator1 : RelationalOperator  Operator=>  OutDataTypeStr=boolean  InputSameDT=off
  Pulse : Outport  VectorParamsAs1DForOutWhenUnconnected=off
  wires:
  Relational Operator1/1 -> Discrete-Time Integrator/2
  Constant1/1 -> Relational Operator1/2
  Compare To Constant/1 -> Pulse/1
  Discrete-Time Integrator/State -> Relational Operator1/1
  Discrete-Time Integrator/1 -> Compare To Constant/1
  Freq/1 -> Discrete-Time Integrator/1

== stateflow chart PV_MPPT_DesktopSim/MPPT and Boost Controllers/Perturb and Observe MPPT1 ==
  state DisableMPPT
    during:
    Vref = VrefCmd;
    Vref_prev = VrefCmd;
  state EnableMPPT
    state Compute_Power
      entry:
      P = V*I;
    state Calculate_Difference
      entry:
      deltaP = P - Pprev;
      deltaV = V - Vprev;
    state Decrement_Vref
      entry:
      Vref = Vref_prev - delV;
    state Increment_Vref
      entry:
      Vref = Vref_prev + delV;
    state Save_PreviousValues
      entry:
      Pprev = P; Vprev = V;
    state Clamp_VrefMax
      entry:
      Vref = VrefMax;
    state Clamp_VrefMin
      entry:
      Vref = VrefMin;
    (default) -> Compute_Power
    (junction 76) -> Compute_Power
    (junction 53) -> (junction 76) : {Vref_prev = Vref;}
    Compute_Power -> Calculate_Difference
    Calculate_Difference -> (junction 13) [order 1] : [deltaP < 0]
    Calculate_Difference -> (junction 14) [order 2] : [deltaP >= 0]
    (junction 13) -> Increment_Vref [order 2] : [deltaV < 0]
    (junction 14) -> Decrement_Vref [order 1] : [deltaV <= 0]
    (junction 13) -> Decrement_Vref [order 1] : [deltaV >= 0]
    (junction 14) -> Increment_Vref [order 2] : [deltaV > 0]
    Decrement_Vref -> Save_PreviousValues
    Increment_Vref -> Save_PreviousValues
    Save_PreviousValues -> (junction 53) [order 3]
    (junction 73) -> (junction 53)
    Save_PreviousValues -> Clamp_VrefMax [order 1] : [Vref >= VrefMax]
    Save_PreviousValues -> Clamp_VrefMin [order 2] : [Vref <= VrefMin]
    Clamp_VrefMax -> (junction 70)
    Clamp_VrefMin -> (junction 50)
    (junction 70) -> (junction 50)
    (junction 50) -> (junction 73)
  (default) -> DisableMPPT
  (junction 91) -> DisableMPPT
  EnableMPPT -> (junction 91) : [MPPT ~= 1]
  DisableMPPT -> EnableMPPT : [MPPT == 1]
  data: P local double =0; k local double =0; Psum local double =0; Vsum local double =0; Vavg local double =0; Pavg local double =0; deltaP local double =0; Pprev local double =0; Vprev local double =0; deltaV local double =0; Vref output double =5; Vref_prev local double =5; VrefMax constant double =28; VrefMin constant double =1; V input double; I input double; VrefCmd input double; MPPT input double; delV input double
  events: event input RISING_EDGE_EVENT

== matlab function PV_MPPT_DesktopSim/MATLAB Function ==
  settings: updateMethod=DISCRETE
  data: Vpv input; Ipv input; ArrayPower parameter; ArrayVoltage parameter; numIrr parameter
function plotPower(Vpv,Ipv, ArrayPower,ArrayVoltage, numIrr)

    persistent irrPlot powerPlot
%     coder.extrinsic('legend');    
    
    if isempty(irrPlot)
        
        idx = 1:find(ArrayPower(:,numIrr) > 0,1,'last')+2;
                        
        figure(1);
        irrPlot = plot(ArrayVoltage(idx),ArrayPower(idx,1:numIrr)); hold on;
        grid on;
        
        xlabel('PV Voltage [V]');
        ylabel('PV Power [W]');
        title('PV Power Output');
        
        powerPlot = plot(Vpv,Vpv*Ipv,'ro'); 
%         legend('50 W/m^2','100 W/m^2','150 W/m^2','200 W/m^2','250 W/m^2','300 W/m^2',...
%             '350 W/m^2','400 W/m^2','450 W/m^2','500 W/m^2','PV Power');
        hold off;
        
    else 
        set(powerPlot,'XData',Vpv,'YData',Vpv*Ipv);
    end
    
end
